simulink model "System_Design_Quadrocopter_Dynamics3"  (Simulink 7.4)
settings: Solver=ode45  StartTime=0.0  StopTime=inf  RelTol=1e-3
values from neighbouring files (symbols this model uses):
  K_ret = place(System.a, System.b, [-18 -10 -9 -5 -7])    [Test_Reglerauslegung.m]    (also in auslegung.m = place(System.a, System.b, [-2 -4 -3]))
  KV = KV'    [Reglerauslegung.m]    (also in Test_Reglerauslegung.m; auslegung.m)
  KvPhi = 0.5    [Test_Reglerauslegung.m]
  KvPsi = 0.08    [Test_Reglerauslegung.m]
  KvTheta = 0.4    [Test_Reglerauslegung.m]
undefined symbols (not defined in the file or in its folder): g, m, Ts
libraries: simulink x13, dspobslib x4, Control_lib x2, Copter_Library x1
(part 1 of 2)
settings Model: Creator=roczit00  LastModifiedBy=Mole
settings DebuggingCC: AlgebraicLoopMsg=none  SolverPrmCheckMsg=none  UnconnectedInputMsg=none  UnconnectedOutputMsg=none  UnconnectedLineMsg=none

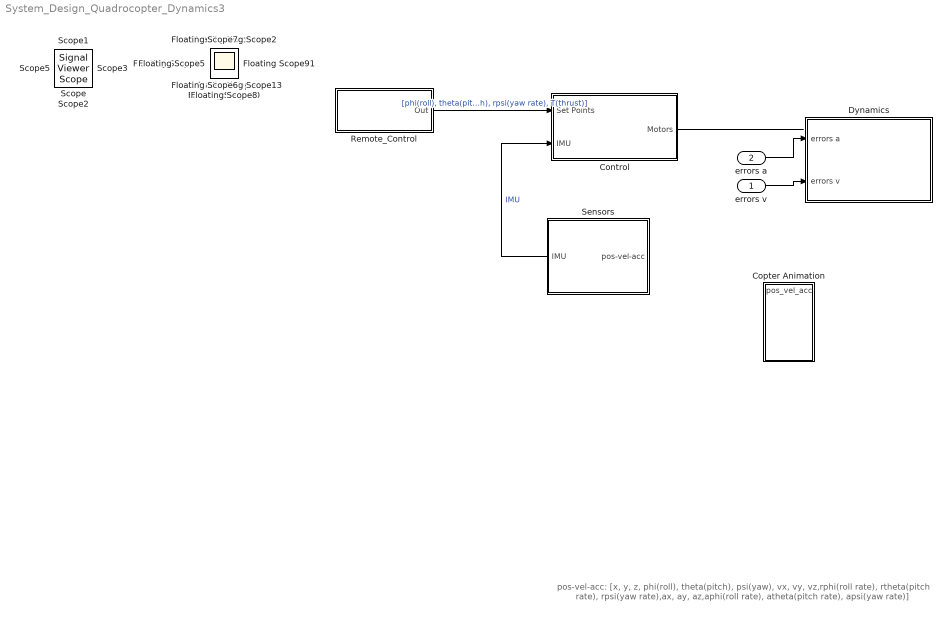
== system System_Design_Quadrocopter_Dynamics3 ==
  note: pos-vel-acc: [x, y, z, phi(roll), theta(pitch), psi(yaw), vx, vy, vz,rphi(roll rate), rtheta(pitch rate), rpsi(yaw rate),ax, ay, az,aphi(roll rate), atheta(pitch rate), apsi(yaw rate)]
  errors v : Inport
  errors a : Inport  Port=2
  Control : Subsystem
  Copter Animation : Subsystem  mask(Quadrocopter Animation){AXES=[-100 100 -100 100 0 100], T_INT=1/25, K_VAR=Feste Position, K_POS=[30 0 6], K_ANGLE=27, A_ON=on, u_phi=on, u_theta=on, u_psi=on, u_x=on, u_y=on, u_z=off}
      mask prompts: AXES "Achsen Grenzen [xmin xmax ymin ymax zmin zmax]"; T_INT "Zeitintervall zwischen Aktualisierungen [s]:"; K_VAR "Kamera Art:"; K_POS "Ort der Kamera [xc yc zc]:"; K_ANGLE "Öffnungswinkel der Kamera [Grad]:"; A_ON "Animation Einschalten:"; u_phi "Use Input phi:"; u_theta "Use Input theta:"; u_psi "Use Input psi:"; u_x "Use Input x:"; u_y "Use Input y:"; u_z "Use Input z:"
      mask help: Erstellt eine 3-D animierte Ansicht eines Quadrocopters.
      mask init:
      | Config.axes = AXES;
      | Config.update = T_INT;
      | Config.camera_view = K_VAR;
      | Config.camera_pos = K_POS;
      | Config.view = K_ANGLE;
      | Config.Animenable = A_ON;
      | Config.phi = u_phi;
      | Config.theta = u_theta;
      | Config.psi = u_psi;
      | Config.x = u_x;
      | Config.y = u_y;
      | Config.z = u_z;
      mask Help:
      | <p>Dieser Block erstellt ein 3 dimensionales Fenster eines Quadrocopters.
      | 
      | <p><H4>Block Eingänge</H4>
      | Der Eingangsvektor bestehend aus:
      | <ul>
      | <li>X-Koordinate - Ort bezogen auf die X-Achse
      | <li>Y-Koordinate - Ort bezogen auf die Y-Achse
      | <li>Z-Koordinate - Ort bezogen auf die Z-Achse
      | <li>Psi - Yaw Drehung um die Z-Achse
      | <li>Phi - Roll Drehen um die Achse in Flugrichtung
      | <li>theta - pitch Neigung in Flugrichtung nach oben bzw. unten
      | </ul></p>
      mask StyleString: edit,edit,popup(Feste Position|Frei bewegbar),edit,edit,checkbox,checkbox,checkbox,checkbox,checkbox,checkbox,checkbox
  Dynamics : Subsystem
  Remote_Control : Subsystem
  Sensors : Subsystem
  Floating Scope{,1..13} (14 alike) : Scope
      Floating Scope settings: Floating=on  YMin=-40  YMax=90
      Floating Scope1 settings: Floating=on
      Floating Scope10 settings: Floating=on  SaveName=ScopeData12
      Floating Scope11 settings: Floating=on  SaveName=ScopeData13
      Floating Scope12 settings: Floating=on  YMin=-2500  YMax=27500  SaveName=ScopeData14
      Floating Scope13 settings: Floating=on  YMin=0  YMax=0.3  SaveName=ScopeData15
      Floating Scope2 settings: Floating=on  YMin=-6000  YMax=2500  SaveName=ScopeData2
      Floating Scope3 settings: Floating=on  SaveName=ScopeData3
      Floating Scope4 settings: Floating=on  SaveName=ScopeData4
      Floating Scope5 settings: Floating=on  YMin=-0.7  YMax=0.8  SaveName=ScopeData5
      Floating Scope6 settings: Floating=on  YMin=-1  YMax=1  SaveName=ScopeData6
      Floating Scope7 settings: Floating=on  YMin=-15  YMax=10  SaveName=ScopeData7
      Floating Scope8 settings: Floating=on  YMax=45  SaveName=ScopeData10
      Floating Scope9 settings: Floating=on  YMin=-7  YMax=9  SaveName=ScopeData11
  Scope{,1..3,5} (5 alike) : SignalViewerScope  IOType=viewer  RefreshTime=0.035000
      Scope settings: YMin=-0.01  YMax=0.1
      Scope2 settings: SaveName=ScopeData2
      Scope3 settings: SaveName=ScopeData3
      Scope5 settings: YMin=0  YMax=275  SaveName=ScopeData4
  wires:
  ? -> Copter Animation/1(pos_vel_acc), Sensors/1(pos-vel-acc)  "pos-vel-acc"
  Sensors/1(IMU) -> Control/2(IMU)  "IMU"
  Remote_Control/1(Out) -> Control/1(Set Points)  "[phi(roll), theta(pitch), rpsi(yaw rate), T(thrust)]"
  errors v/1 -> Dynamics/2(errors v)
  Control/1(Motors) -> ?
  errors a/1 -> Dynamics/1(errors a)

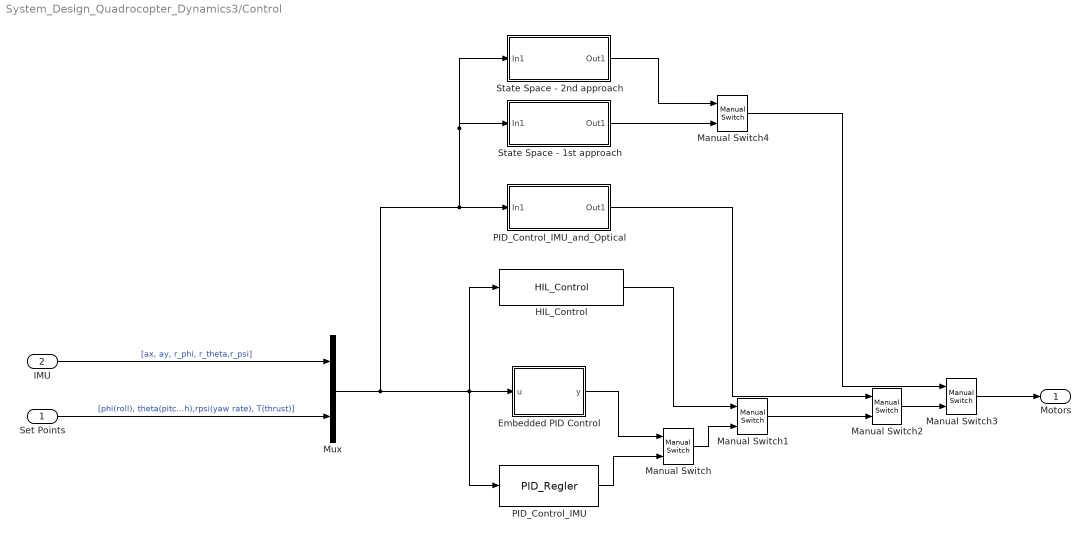
== system System_Design_Quadrocopter_Dynamics3/Control ==
  Set Points : Inport  PortDimensions=4  DataType=double  OutDataTypeStr=double
  IMU : Inport  Port=2
  Embedded PID Control : Stateflow chart  TreatAsAtomicUnit=on
  HIL_Control : Control_lib/HIL_Control  enabled=off
  Manual Switch{,2..4} (4 alike) : simulink/Signal Routing/Manual Switch  SystemSampleTime=-1  sw=1  action=0  varsize=off
  Manual Switch1 : simulink/Signal Routing/Manual Switch  SystemSampleTime=-1  sw=0  action=0  varsize=off
  Mux : Mux  Inputs=2
  PID_Control_IMU : Control_lib/PID_Regler  SystemSampleTime=-1
  PID_Control_IMU_and_Optical : Subsystem  AncestorBlock=Control_lib/PID_Regler
  State Space - 1st approach : Subsystem
  State Space - 2nd approach : Subsystem
  Motors : Outport  PortDimensions=4
  wires:
  IMU/1 -> Mux/1  "[ax, ay, r_phi, r_theta,r_psi]"
  Set Points/1 -> Mux/2  "[phi(roll), theta(pitch),rpsi(yaw rate), T(thrust)]"
  PID_Control_IMU/1 -> Manual Switch/2
  Mux/1 -> PID_Control_IMU/1, HIL_Control/1, Embedded PID Control/1(u), PID_Control_IMU_and_Optical/1(In1), State Space - 1st approach/1(In1), State Space - 2nd approach/1(In1)
  Manual Switch/1 -> Manual Switch1/2
  Manual Switch1/1 -> Manual Switch2/2
  Embedded PID Control/1(y) -> Manual Switch/1
  HIL_Control/1 -> Manual Switch1/1
  PID_Control_IMU_and_Optical/1(Out1) -> Manual Switch2/1
  Manual Switch2/1 -> Manual Switch3/2
  Manual Switch3/1 -> Motors/1
  Manual Switch4/1 -> Manual Switch3/1
  State Space - 1st approach/1(Out1) -> Manual Switch4/2
  State Space - 2nd approach/1(Out1) -> Manual Switch4/1

== system System_Design_Quadrocopter_Dynamics3/Copter Animation ==
  pos_vel_acc : Inport  PortDimensions=19
  S-Function : S-Function  FunctionName=Copter_Animation  Parameters=Config  EnableBusSupport=off
  Selector2 : Selector  InputPortWidth=19  IndexOptions=Index vector (dialog)  Indices=[1 2 3 4 5 6]  OutputSizes=1
  wires:
  pos_vel_acc/1 -> Selector2/1
  Selector2/1 -> S-Function/1

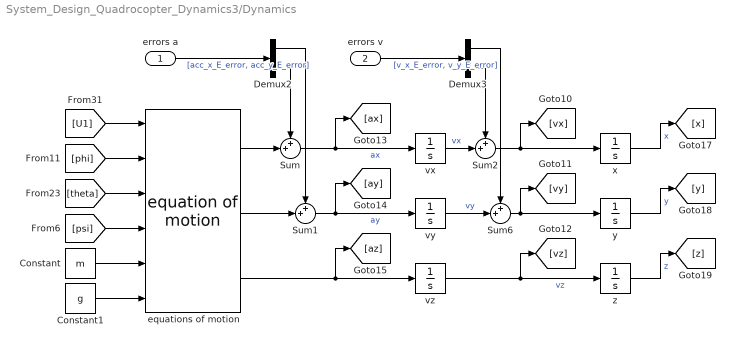
== system System_Design_Quadrocopter_Dynamics3/Dynamics ==
  errors a : Inport
  errors v : Inport  Port=2
  Constant : Constant  Value=m
  Constant1 : Constant  Value=g
  Demux2 : Demux  Outputs=2
  Demux3 : Demux  Outputs=2
  Sum{,1..2,6} (4 alike) : Sum  Inputs=++|
  equations of motion : Copter_Library/equation of motion  SystemSampleTime=-1
  vx : Integrator
  vy : Integrator
  vz : Integrator
  x : Integrator
  y : Integrator
  z : Integrator
  wires:
  errors a/1 -> Demux2/1  "[acc_x_E_error, acc_y_E_error]"
  vz/1 -> [vz], z/1  "vz"
  Demux2/2 -> Sum/1
  Demux2/1 -> Sum1/1
  equations of motion/3 -> [az], vz/1
  equations of motion/2 -> Sum1/2
  equations of motion/1 -> Sum/2
  [phi] -> equations of motion/2
  [theta] -> equations of motion/3
  [psi] -> equations of motion/4
  Constant/1 -> equations of motion/5
  Constant1/1 -> equations of motion/6
  errors v/1 -> Demux3/1  "[v_x_E_error, v_y_E_error]"
  Demux3/2 -> Sum2/1
  Demux3/1 -> Sum6/1
  vx/1 -> Sum2/2  "vx"
  Sum2/1 -> [vx], x/1
  vy/1 -> Sum6/2  "vy"
  Sum6/1 -> y/1, [vy]
  z/1 -> [z]  "z"
  y/1 -> [y]  "y"
  x/1 -> [x]  "x"
  Sum1/1 -> vy/1, [ay]  "ay"
  Sum/1 -> vx/1, [ax]  "ax"
  [U1] -> equations of motion/1

== system System_Design_Quadrocopter_Dynamics3/Remote_Control ==
  3D-Mouse : simulink/Signal Routing/Manual Switch  SystemSampleTime=-1  sw=0  action=0  varsize=off
  Allow 3D Mouse : dspobslib/DSP Constant  SystemSampleTime=-1  Value=1  SampleMode=Discrete  discreteOutput=Sample-based  continuousOutput=Sample-based  sampTime=inf  framePeriod=2  dataType=boolean  isSigned=on  wordLen=16  udDataType=sfix(16)  fracBitsMode=Best precision  numFracBits=15  InterpretAs1D=-inf  Ts=-inf  FramebasedOutput=-inf
  Disable 3D Mouse : dspobslib/DSP Constant  SystemSampleTime=-1  Value=0  SampleMode=Discrete  discreteOutput=Sample-based  continuousOutput=Sample-based  sampTime=inf  framePeriod=2  dataType=boolean  isSigned=on  wordLen=16  udDataType=sfix(16)  fracBitsMode=Best precision  numFracBits=15  InterpretAs1D=-inf  Ts=-inf  FramebasedOutput=-inf
  Manual Switch2 : simulink/Signal Routing/Manual Switch  SystemSampleTime=-1  sw=1  action=0  varsize=off
  Remote_Control_3d_mouse : Subsystem  AncestorBlock=Remote_Control_Library/Remote_Control_3d_mouse
  Remote_Control_Pitch_stimuli1 : Subsystem  AncestorBlock=Remote_Control_Library/Remote_Control_Pitch_stimuli
  Out : Outport
  wires:
  Remote_Control_Pitch_stimuli1/1(Out) -> Manual Switch2/1
  Manual Switch2/1 -> Out/1
  Allow 3D Mouse/1 -> 3D-Mouse/1
  Disable 3D Mouse/1 -> 3D-Mouse/2
  3D-Mouse/1 -> Remote_Control_3d_mouse/Enable
  Remote_Control_3d_mouse/1(Out1) -> Manual Switch2/2

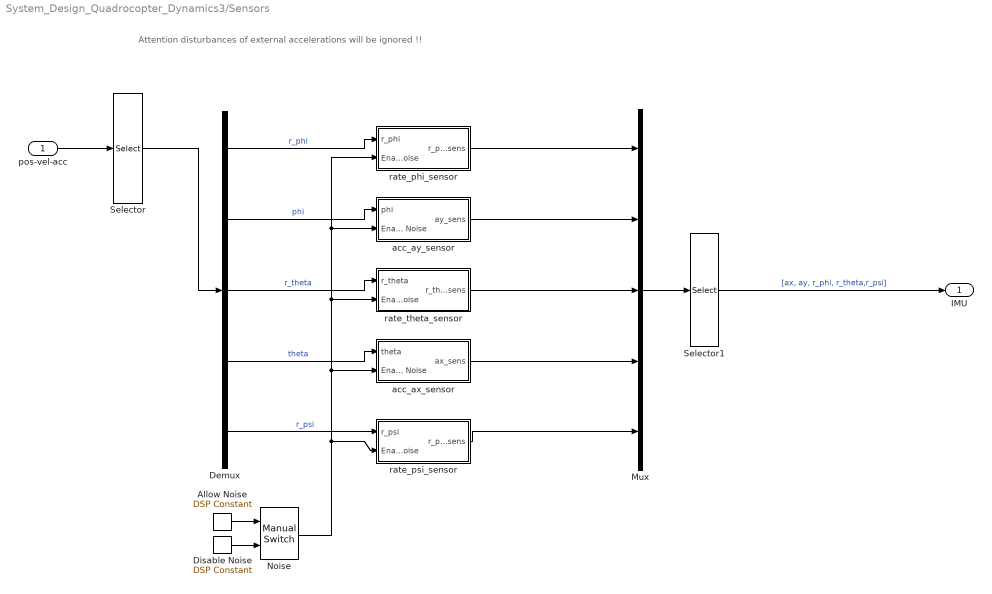
== system System_Design_Quadrocopter_Dynamics3/Sensors ==
  note: Attention disturbances of external accelerations will be ignored !!
  pos-vel-acc : Inport  PortDimensions=19
  Allow Noise : dspobslib/DSP Constant  SystemSampleTime=-1  Value=1  SampleMode=Discrete  discreteOutput=Sample-based  continuousOutput=Sample-based  sampTime=inf  framePeriod=2  dataType=boolean  isSigned=on  wordLen=16  udDataType=sfix(16)  fracBitsMode=Best precision  numFracBits=15  InterpretAs1D=-inf  Ts=-inf  FramebasedOutput=-inf
  Demux : Demux  Outputs=5
  Disable Noise : dspobslib/DSP Constant  SystemSampleTime=-1  Value=0  SampleMode=Discrete  discreteOutput=Sample-based  continuousOutput=Sample-based  sampTime=inf  framePeriod=2  dataType=boolean  isSigned=on  wordLen=16  udDataType=sfix(16)  fracBitsMode=Best precision  numFracBits=15  InterpretAs1D=-inf  Ts=-inf  FramebasedOutput=-inf
  Mux : Mux  Inputs=5
  Noise : simulink/Signal Routing/Manual Switch  SystemSampleTime=-1  sw=1  action=0  varsize=off
  Selector : Selector  InputPortWidth=19  IndexOptions=Index vector (dialog)  Indices=[10 4 11 5 12]  OutputSizes=1
  Selector1 : Selector  InputPortWidth=5  IndexOptions=Index vector (dialog)  Indices=[4 2 1 3 5]  OutputSizes=1
  acc_ax_sensor : Subsystem
  acc_ay_sensor : Subsystem
  rate_phi_sensor : Subsystem
  rate_psi_sensor : Subsystem
  rate_theta_sensor : Subsystem
  IMU : Outport
  wires:
  pos-vel-acc/1 -> Selector/1
  Selector/1 -> Demux/1
  rate_phi_sensor/1(r_phi_sens) -> Mux/1
  acc_ay_sensor/1(ay_sens) -> Mux/2
  rate_theta_sensor/1(r_theta_sens) -> Mux/3
  acc_ax_sensor/1(ax_sens) -> Mux/4
  rate_psi_sensor/1(r_psi_sens) -> Mux/5
  Demux/1 -> rate_phi_sensor/1(r_phi)  "r_phi"
  Demux/2 -> acc_ay_sensor/1(phi)  "phi"
  Demux/3 -> rate_theta_sensor/1(r_theta)  "r_theta"
  Demux/4 -> acc_ax_sensor/1(theta)  "theta"
  Demux/5 -> rate_psi_sensor/1(r_psi)  "r_psi"
  Mux/1 -> Selector1/1
  Selector1/1 -> IMU/1  "[ax, ay, r_phi, r_theta,r_psi]"
  Allow Noise/1 -> Noise/1
  Disable Noise/1 -> Noise/2
  Noise/1 -> rate_psi_sensor/2(Enable Noise), acc_ax_sensor/2(Enable Noise), rate_theta_sensor/2(Enable Noise), acc_ay_sensor/2(Enable Noise), rate_phi_sensor/2(Enable Noise)

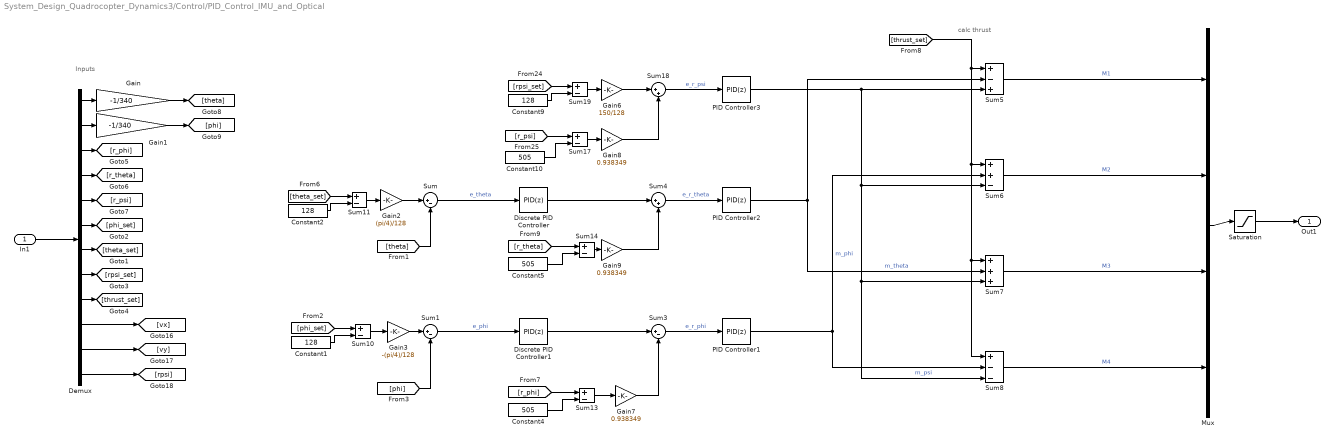
== system System_Design_Quadrocopter_Dynamics3/Control/PID_Control_IMU_and_Optical ==
  note: calc thrust
  note: Inputs
  In1 : Inport  OutDataType=fixdt(1, 16)  OutScaling=2^0
  Constant1 : Constant  Value=128  OutDataType=fixdt(1, 16)  OutScaling=2^0
  Constant10 : Constant  Value=505  OutDataType=fixdt(1, 16)  OutScaling=2^0
  Constant2 : Constant  Value=128  OutDataType=fixdt(1, 16)  OutScaling=2^0
  Constant4 : Constant  Value=505  OutDataType=fixdt(1, 16)  OutScaling=2^0
  Constant5 : Constant  Value=505  OutDataType=fixdt(1, 16)  OutScaling=2^0
  Constant9 : Constant  Value=128  OutDataType=fixdt(1, 16)  OutScaling=2^0
  Demux : Demux  Outputs=12
  Discrete PID Controller : simulink/Continuous/PID Controller  DialogController=pidpack.PIDConfig.pidDDGCreate  DialogControllerArgs=DataTag0  SystemSampleTime=-1  Controller=PID  TimeDomain=Discrete-time  SampleTime=Ts  IntegratorMethod=Forward Euler  FilterMethod=Forward Euler  Form=Ideal  P=150  I=0.5  D=0  N=0  InitialConditionSource=internal  InitialConditionForIntegrator=0  InitialConditionForFilter=0  ExternalReset=none  ZeroCross=off  LimitOutput=off  UpperSaturationLimit=inf  LowerSaturationLimit=-inf  LinearizeAsGain=off  AntiWindupMode=none  Kb=1  TrackingMode=off  Kt=1  PParamMin=[]  PParamMax=[]  IParamMin=[]  IParamMax=[]  DParamMin=[]  DParamMax=[]  NParamMin=[]  NParamMax=[]  KbParamMin=[]  KbParamMax=[]  KtParamMin=[]  KtParamMax=[]  POutMin=[]  POutMax=[]  IOutMin=[]  IOutMax=[]  DOutMin=[]  DOutMax=[]  NOutMin=[]  NOutMax=[]  KbOutMin=[]  KbOutMax=[]  KtOutMin=[]  KtOutMax=[]  IntegratorOutMin=[]  IntegratorOutMax=[]  FilterOutMin=[]  FilterOutMax=[]  SumOutMin=[]  SumOutMax=[]  SumI1OutMin=[]  SumI1OutMax=[]  SumI2OutMin=[]  SumI2OutMax=[]  SumI3OutMin=[]  SumI3OutMax=[]  SumDOutMin=[]  SumDOutMax=[]  SaturationOutMin=[]  SaturationOutMax=[]  IntegratorContinuousStateAttributes=''  IntegratorStateMustResolveToSignalObject=off  IntegratorRTWStateStorageClass=Auto  FilterContinuousStateAttributes=''  FilterStateMustResolveToSignalObject=off  FilterRTWStateStorageClass=Auto
  Discrete PID Controller1 : simulink/Continuous/PID Controller  DialogController=pidpack.PIDConfig.pidDDGCreate  DialogControllerArgs=DataTag1  SystemSampleTime=-1  Controller=PID  TimeDomain=Discrete-time  SampleTime=Ts  IntegratorMethod=Forward Euler  FilterMethod=Forward Euler  Form=Ideal  P=150  I=0.5  D=0  N=0  InitialConditionSource=internal  InitialConditionForIntegrator=0  InitialConditionForFilter=0  ExternalReset=none  ZeroCross=off  LimitOutput=off  UpperSaturationLimit=inf  LowerSaturationLimit=-inf  LinearizeAsGain=off  AntiWindupMode=none  Kb=1  TrackingMode=off  Kt=1  PParamMin=[]  PParamMax=[]  IParamMin=[]  IParamMax=[]  DParamMin=[]  DParamMax=[]  NParamMin=[]  NParamMax=[]  KbParamMin=[]  KbParamMax=[]  KtParamMin=[]  KtParamMax=[]  POutMin=[]  POutMax=[]  IOutMin=[]  IOutMax=[]  DOutMin=[]  DOutMax=[]  NOutMin=[]  NOutMax=[]  KbOutMin=[]  KbOutMax=[]  KtOutMin=[]  KtOutMax=[]  IntegratorOutMin=[]  IntegratorOutMax=[]  FilterOutMin=[]  FilterOutMax=[]  SumOutMin=[]  SumOutMax=[]  SumI1OutMin=[]  SumI1OutMax=[]  SumI2OutMin=[]  SumI2OutMax=[]  SumI3OutMin=[]  SumI3OutMax=[]  SumDOutMin=[]  SumDOutMax=[]  SaturationOutMin=[]  SaturationOutMax=[]  IntegratorContinuousStateAttributes=''  IntegratorStateMustResolveToSignalObject=off  IntegratorRTWStateStorageClass=Auto  FilterContinuousStateAttributes=''  FilterStateMustResolveToSignalObject=off  FilterRTWStateStorageClass=Auto
  Gain : Gain  Gain=-1/340  ParameterDataType=fixdt(1, 16)  ParameterScaling=2^0  OutDataType=fixdt(1, 16)  OutScaling=2^0
  Gain1 : Gain  Gain=-1/340  ParameterDataType=fixdt(1, 16)  ParameterScaling=2^0  OutDataType=fixdt(1, 16)  OutScaling=2^0
  Gain2 : Gain  Gain=(pi/4)/128  ParameterDataType=fixdt(1, 16)  ParameterScaling=2^0  OutDataType=fixdt(1, 16)  OutScaling=2^0
  Gain3 : Gain  Gain=-(pi/4)/128  ParameterDataType=fixdt(1, 16)  ParameterScaling=2^0  OutDataType=fixdt(1, 16)  OutScaling=2^0
  Gain6 : Gain  Gain=150/128  ParameterDataType=fixdt(1, 16)  ParameterScaling=2^0  OutDataType=fixdt(1, 16)  OutScaling=2^0
  Gain7 : Gain  Gain=0.938349  ParameterDataType=fixdt(1, 16)  ParameterScaling=2^0  OutDataType=fixdt(1, 16)  OutScaling=2^0
  Gain8 : Gain  Gain=0.938349  ParameterDataType=fixdt(1, 16)  ParameterScaling=2^0  OutDataType=fixdt(1, 16)  OutScaling=2^0
  Gain9 : Gain  Gain=0.938349  ParameterDataType=fixdt(1, 16)  ParameterScaling=2^0  OutDataType=fixdt(1, 16)  OutScaling=2^0
  Mux : Mux
  PID Controller1 : simulink/Continuous/PID Controller  DialogController=pidpack.PIDConfig.pidDDGCreate  DialogControllerArgs=DataTag2  SystemSampleTime=-1  Controller=PID  TimeDomain=Discrete-time  SampleTime=Ts  IntegratorMethod=Forward Euler  FilterMethod=Forward Euler  Form=Ideal  P=60  I=0.5  D=0  N=0  InitialConditionSource=internal  InitialConditionForIntegrator=0  InitialConditionForFilter=0  ExternalReset=none  ZeroCross=off  LimitOutput=off  UpperSaturationLimit=inf  LowerSaturationLimit=-inf  LinearizeAsGain=off  AntiWindupMode=none  Kb=1  TrackingMode=off  Kt=1  PParamMin=[]  PParamMax=[]  IParamMin=[]  IParamMax=[]  DParamMin=[]  DParamMax=[]  NParamMin=[]  NParamMax=[]  KbParamMin=[]  KbParamMax=[]  KtParamMin=[]  KtParamMax=[]  POutMin=[]  POutMax=[]  IOutMin=[]  IOutMax=[]  DOutMin=[]  DOutMax=[]  NOutMin=[]  NOutMax=[]  KbOutMin=[]  KbOutMax=[]  KtOutMin=[]  KtOutMax=[]  IntegratorOutMin=[]  IntegratorOutMax=[]  FilterOutMin=[]  FilterOutMax=[]  SumOutMin=[]  SumOutMax=[]  SumI1OutMin=[]  SumI1OutMax=[]  SumI2OutMin=[]  SumI2OutMax=[]  SumI3OutMin=[]  SumI3OutMax=[]  SumDOutMin=[]  SumDOutMax=[]  SaturationOutMin=[]  SaturationOutMax=[]  IntegratorContinuousStateAttributes=''  IntegratorStateMustResolveToSignalObject=off  IntegratorRTWStateStorageClass=Auto  FilterContinuousStateAttributes=''  FilterStateMustResolveToSignalObject=off  FilterRTWStateStorageClass=Auto
  PID Controller2 : simulink/Continuous/PID Controller  DialogController=pidpack.PIDConfig.pidDDGCreate  DialogControllerArgs=DataTag3  SystemSampleTime=-1  Controller=PID  TimeDomain=Discrete-time  SampleTime=Ts  IntegratorMethod=Forward Euler  FilterMethod=Forward Euler  Form=Ideal  P=60  I=0.5  D=0  N=0  InitialConditionSource=internal  InitialConditionForIntegrator=0  InitialConditionForFilter=0  ExternalReset=none  ZeroCross=off  LimitOutput=off  UpperSaturationLimit=inf  LowerSaturationLimit=-inf  LinearizeAsGain=off  AntiWindupMode=none  Kb=1  TrackingMode=off  Kt=1  PParamMin=[]  PParamMax=[]  IParamMin=[]  IParamMax=[]  DParamMin=[]  DParamMax=[]  NParamMin=[]  NParamMax=[]  KbParamMin=[]  KbParamMax=[]  KtParamMin=[]  KtParamMax=[]  POutMin=[]  POutMax=[]  IOutMin=[]  IOutMax=[]  DOutMin=[]  DOutMax=[]  NOutMin=[]  NOutMax=[]  KbOutMin=[]  KbOutMax=[]  KtOutMin=[]  KtOutMax=[]  IntegratorOutMin=[]  IntegratorOutMax=[]  FilterOutMin=[]  FilterOutMax=[]  SumOutMin=[]  SumOutMax=[]  SumI1OutMin=[]  SumI1OutMax=[]  SumI2OutMin=[]  SumI2OutMax=[]  SumI3OutMin=[]  SumI3OutMax=[]  SumDOutMin=[]  SumDOutMax=[]  SaturationOutMin=[]  SaturationOutMax=[]  IntegratorContinuousStateAttributes=''  IntegratorStateMustResolveToSignalObject=off  IntegratorRTWStateStorageClass=Auto  FilterContinuousStateAttributes=''  FilterStateMustResolveToSignalObject=off  FilterRTWStateStorageClass=Auto
  PID Controller3 : simulink/Continuous/PID Controller  DialogController=pidpack.PIDConfig.pidDDGCreate  DialogControllerArgs=DataTag4  SystemSampleTime=-1  Controller=PID  TimeDomain=Discrete-time  SampleTime=Ts  IntegratorMethod=Forward Euler  FilterMethod=Forward Euler  Form=Ideal  P=60  I=0.5  D=0  N=0  InitialConditionSource=internal  InitialConditionForIntegrator=0  InitialConditionForFilter=0  ExternalReset=none  ZeroCross=off  LimitOutput=off  UpperSaturationLimit=inf  LowerSaturationLimit=-inf  LinearizeAsGain=off  AntiWindupMode=none  Kb=1  TrackingMode=off  Kt=1  PParamMin=[]  PParamMax=[]  IParamMin=[]  IParamMax=[]  DParamMin=[]  DParamMax=[]  NParamMin=[]  NParamMax=[]  KbParamMin=[]  KbParamMax=[]  KtParamMin=[]  KtParamMax=[]  POutMin=[]  POutMax=[]  IOutMin=[]  IOutMax=[]  DOutMin=[]  DOutMax=[]  NOutMin=[]  NOutMax=[]  KbOutMin=[]  KbOutMax=[]  KtOutMin=[]  KtOutMax=[]  IntegratorOutMin=[]  IntegratorOutMax=[]  FilterOutMin=[]  FilterOutMax=[]  SumOutMin=[]  SumOutMax=[]  SumI1OutMin=[]  SumI1OutMax=[]  SumI2OutMin=[]  SumI2OutMax=[]  SumI3OutMin=[]  SumI3OutMax=[]  SumDOutMin=[]  SumDOutMax=[]  SaturationOutMin=[]  SaturationOutMax=[]  IntegratorContinuousStateAttributes=''  IntegratorStateMustResolveToSignalObject=off  IntegratorRTWStateStorageClass=Auto  FilterContinuousStateAttributes=''  FilterStateMustResolveToSignalObject=off  FilterRTWStateStorageClass=Auto
  Saturation : Saturate  UpperLimit=255  LowerLimit=0  OutDataType=fixdt(1, 16)  OutScaling=2^0
  Sum : Sum  Inputs=|+-  OutDataType=fixdt(1, 16)  OutScaling=2^0
  Sum1 : Sum  Inputs=|+-  OutDataType=fixdt(1, 16)  OutScaling=2^0
  Sum{10..11,13..14,17,19} (6 alike) : Sum  Inputs=+-  OutDataType=fixdt(1, 16)  OutScaling=2^0
  Sum18 : Sum  Inputs=|++  OutDataType=fixdt(1, 16)  OutScaling=2^0
  Sum3 : Sum  Inputs=|+-  OutDataType=fixdt(1, 16)  OutScaling=2^0
  Sum4 : Sum  Inputs=|++  OutDataType=fixdt(1, 16)  OutScaling=2^0
  Sum5 : Sum  Inputs=+-+  OutDataType=fixdt(1, 16)  OutScaling=2^0
  Sum6 : Sum  Inputs=++-  OutDataType=fixdt(1, 16)  OutScaling=2^0
  Sum7 : Sum  Inputs=+++  OutDataType=fixdt(1, 16)  OutScaling=2^0
  Sum8 : Sum  Inputs=+--  OutDataType=fixdt(1, 16)  OutScaling=2^0
  Out1 : Outport  OutDataType=fixdt(1, 16)  OutScaling=2^0
  wires:
  Sum14/1 -> Gain9/1
  Gain9/1 -> Sum4/2
  Sum13/1 -> Gain7/1
  Gain3/1 -> Sum1/1
  Gain2/1 -> Sum/1
  Sum11/1 -> Gain2/1
  Sum10/1 -> Gain3/1
  [r_theta] -> Sum14/1
  Constant5/1 -> Sum14/2
  [r_phi] -> Sum13/1
  Constant4/1 -> Sum13/2
  Constant2/1 -> Sum11/2
  [theta_set] -> Sum11/1
  Constant1/1 -> Sum10/2
  [phi_set] -> Sum10/1
  Saturation/1 -> Out1/1
  Mux/1 -> Saturation/1
  [thrust_set] -> Sum8/1, Sum7/1, Sum6/1, Sum5/1
  PID Controller1/1 -> Sum6/2, Sum8/2  "m_phi"
  Sum6/1 -> Mux/2  "M2"
  Sum7/1 -> Mux/3  "M3"
  Sum8/1 -> Mux/4  "M4"
  Sum5/1 -> Mux/1  "M1"
  Sum4/1 -> PID Controller2/1  "e_r_theta"
  Sum3/1 -> PID Controller1/1  "e_r_phi"
  Sum1/1 -> Discrete PID Controller1/1  "e_phi"
  [phi] -> Sum1/2
  Sum/1 -> Discrete PID Controller/1  "e_theta"
  [theta] -> Sum/2
  Gain1/1 -> [phi]
  Gain/1 -> [theta]
  Demux/9 -> [thrust_set]
  Demux/8 -> [rpsi_set]
  Demux/7 -> [theta_set]
  Demux/6 -> [phi_set]
  Demux/5 -> [r_psi]
  Demux/4 -> [r_theta]
  Demux/3 -> [r_phi]
  Demux/1 -> Gain/1
  Demux/2 -> Gain1/1
  In1/1 -> Demux/1
  Demux/10 -> [vx]
  Demux/11 -> [vy]
  Demux/12 -> [rpsi]
  Gain8/1 -> Sum18/2
  Sum17/1 -> Gain8/1
  Gain6/1 -> Sum18/1
  Sum19/1 -> Gain6/1
  Constant10/1 -> Sum17/2
  [r_psi] -> Sum17/1
  Constant9/1 -> Sum19/2
  [rpsi_set] -> Sum19/1
  Sum18/1 -> PID Controller3/1  "e_r_psi"
  Discrete PID Controller1/1 -> Sum3/1
  Discrete PID Controller/1 -> Sum4/1
  Gain7/1 -> Sum3/2
  PID Controller3/1 -> Sum5/3, Sum6/3, Sum7/3, Sum8/3  "m_psi"
  PID Controller2/1 -> Sum7/2, Sum5/2  "m_theta"

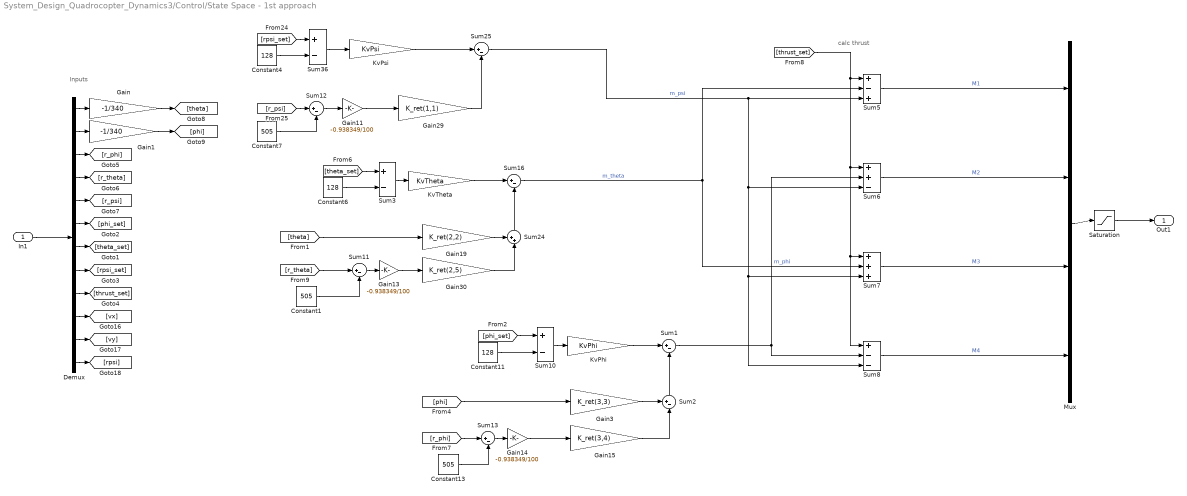
== system System_Design_Quadrocopter_Dynamics3/Control/State Space - 1st approach ==
  note: calc thrust
  note: Inputs
  In1 : Inport  OutDataType=fixdt(1, 16)  OutScaling=2^0
  Constant1 : Constant  Value=505  OutDataType=fixdt(1, 16)  OutScaling=2^0
  Constant11 : Constant  Value=128  OutDataType=fixdt(1, 16)  OutScaling=2^0
  Constant13 : Constant  Value=505  OutDataType=fixdt(1, 16)  OutScaling=2^0
  Constant4 : Constant  Value=128  OutDataType=fixdt(1, 16)  OutScaling=2^0
  Constant6 : Constant  Value=128  OutDataType=fixdt(1, 16)  OutScaling=2^0
  Constant7 : Constant  Value=505  OutDataType=fixdt(1, 16)  OutScaling=2^0
  Demux : Demux  Outputs=12
  Gain : Gain  Gain=-1/340  ParameterDataType=fixdt(1, 16)  ParameterScaling=2^0  OutDataType=fixdt(1, 16)  OutScaling=2^0
  Gain1 : Gain  Gain=-1/340  ParameterDataType=fixdt(1, 16)  ParameterScaling=2^0  OutDataType=fixdt(1, 16)  OutScaling=2^0
  Gain11 : Gain  Gain=-0.938349/100  ParameterDataType=fixdt(1, 16)  ParameterScaling=2^0  OutDataType=fixdt(1, 16)  OutScaling=2^0
  Gain13 : Gain  Gain=-0.938349/100  ParameterDataType=fixdt(1, 16)  ParameterScaling=2^0  OutDataType=fixdt(1, 16)  OutScaling=2^0
  Gain14 : Gain  Gain=-0.938349/100  ParameterDataType=fixdt(1, 16)  ParameterScaling=2^0  OutDataType=fixdt(1, 16)  OutScaling=2^0
  Gain15 : Gain  Gain=K_ret(3,4)  ParameterDataType=fixdt(1, 16)  ParameterScaling=2^0  OutDataType=fixdt(1, 16)  OutScaling=2^0
  Gain19 : Gain  Gain=K_ret(2,2)  ParameterDataType=fixdt(1, 16)  ParameterScaling=2^0  OutDataType=fixdt(1, 16)  OutScaling=2^0
  Gain29 : Gain  Gain=K_ret(1,1)  ParameterDataType=fixdt(1, 16)  ParameterScaling=2^0  OutDataType=fixdt(1, 16)  OutScaling=2^0
  Gain3 : Gain  Gain=K_ret(3,3)  ParameterDataType=fixdt(1, 16)  ParameterScaling=2^0  OutDataType=fixdt(1, 16)  OutScaling=2^0
  Gain30 : Gain  Gain=K_ret(2,5)  ParameterDataType=fixdt(1, 16)  ParameterScaling=2^0  OutDataType=fixdt(1, 16)  OutScaling=2^0
  KvPhi : Gain  Gain=KvPhi  ParameterDataType=fixdt(1, 16)  ParameterScaling=2^0  OutDataType=fixdt(1, 16)  OutScaling=2^0
  KvPsi : Gain  Gain=KvPsi  ParameterDataType=fixdt(1, 16)  ParameterScaling=2^0  OutDataType=fixdt(1, 16)  OutScaling=2^0
  KvTheta : Gain  Gain=KvTheta  ParameterDataType=fixdt(1, 16)  ParameterScaling=2^0  OutDataType=fixdt(1, 16)  OutScaling=2^0
  Mux : Mux
  Saturation : Saturate  UpperLimit=255  LowerLimit=0  OutDataType=fixdt(1, 16)  OutScaling=2^0
  Sum{1,11..13,16,25} (6 alike) : Sum  Inputs=|+-  OutDataType=fixdt(1, 16)  OutScaling=2^0
  Sum10 : Sum  Inputs=+-  OutDataType=fixdt(1, 16)  OutScaling=2^0
  Sum2 : Sum  Inputs=+-|  OutDataType=fixdt(1, 16)  OutScaling=2^0
  Sum24 : Sum  Inputs=++|  OutDataType=fixdt(1, 16)  OutScaling=2^0
  Sum3 : Sum  Inputs=+-  OutDataType=fixdt(1, 16)  OutScaling=2^0
  Sum36 : Sum  Inputs=+-  OutDataType=fixdt(1, 16)  OutScaling=2^0
  Sum5 : Sum  Inputs=+-+  OutDataType=fixdt(1, 16)  OutScaling=2^0
  Sum6 : Sum  Inputs=++-  OutDataType=fixdt(1, 16)  OutScaling=2^0
  Sum7 : Sum  Inputs=+++  OutDataType=fixdt(1, 16)  OutScaling=2^0
  Sum8 : Sum  Inputs=+--  OutDataType=fixdt(1, 16)  OutScaling=2^0
  Out1 : Outport  OutDataType=fixdt(1, 16)  OutScaling=2^0
  wires:
  Saturation/1 -> Out1/1
  Mux/1 -> Saturation/1
  [thrust_set] -> Sum8/1, Sum7/1, Sum6/1, Sum5/1
  Sum1/1 -> Sum6/2, Sum8/2  "m_phi"
  Sum6/1 -> Mux/2  "M2"
  Sum7/1 -> Mux/3  "M3"
  Sum8/1 -> Mux/4  "M4"
  Sum5/1 -> Mux/1  "M1"
  Gain1/1 -> [phi]
  Gain/1 -> [theta]
  Demux/9 -> [thrust_set]
  Demux/8 -> [rpsi_set]
  Demux/7 -> [theta_set]
  Demux/6 -> [phi_set]
  Demux/5 -> [r_psi]
  Demux/4 -> [r_theta]
  Demux/3 -> [r_phi]
  Demux/1 -> Gain/1
  Demux/2 -> Gain1/1
  In1/1 -> Demux/1
  Demux/10 -> [vx]
  Demux/11 -> [vy]
  Demux/12 -> [rpsi]
  Sum25/1 -> Sum5/3, Sum6/3, Sum7/3, Sum8/3  "m_psi"
  Sum16/1 -> Sum7/2, Sum5/2  "m_theta"
  Sum2/1 -> Sum1/2
  [r_phi] -> Sum13/1
  Sum10/1 -> KvPhi/1
  Gain3/1 -> Sum2/1
  [phi] -> Gain3/1
  Sum13/1 -> Gain14/1
  Constant13/1 -> Sum13/2
  Gain14/1 -> Gain15/1
  Gain15/1 -> Sum2/2
  KvPhi/1 -> Sum1/1
  Constant11/1 -> Sum10/2
  [phi_set] -> Sum10/1
  KvTheta/1 -> Sum16/1
  Sum24/1 -> Sum16/2
  Sum3/1 -> KvTheta/1
  Gain30/1 -> Sum24/2
  Gain19/1 -> Sum24/1
  [theta] -> Gain19/1
  Gain13/1 -> Gain30/1
  Sum11/1 -> Gain13/1
  Constant1/1 -> Sum11/2
  [r_theta] -> Sum11/1
  [theta_set] -> Sum3/1
  Constant6/1 -> Sum3/2
  KvPsi/1 -> Sum25/1
  Gain29/1 -> Sum25/2
  Sum36/1 -> KvPsi/1
  Gain11/1 -> Gain29/1
  Sum12/1 -> Gain11/1
  [r_psi] -> Sum12/1
  Constant4/1 -> Sum36/2
  [rpsi_set] -> Sum36/1
  Constant7/1 -> Sum12/2

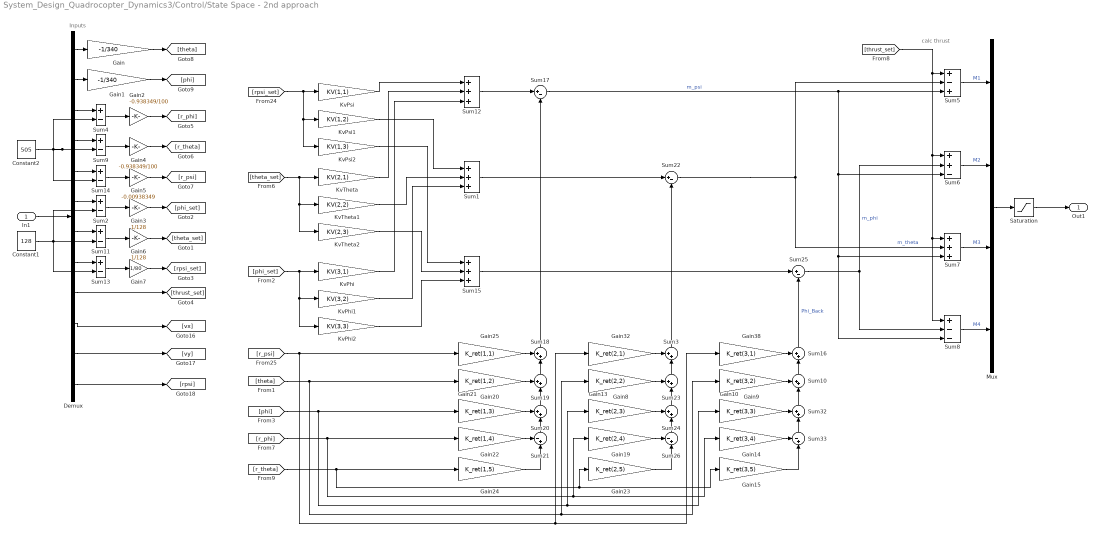
== system System_Design_Quadrocopter_Dynamics3/Control/State Space - 2nd approach ==
  note: calc thrust
  note: Inputs
  In1 : Inport  OutDataType=fixdt(1, 16)  OutScaling=2^0
  Constant1 : Constant  Value=128  OutDataType=fixdt(1, 16)  OutScaling=2^0
  Constant2 : Constant  Value=505  OutDataType=fixdt(1, 16)  OutScaling=2^0
  Demux : Demux  Outputs=12
  Gain : Gain  Gain=-1/340  ParameterDataType=fixdt(1, 16)  ParameterScaling=2^0  OutDataType=fixdt(1, 16)  OutScaling=2^0
  Gain1 : Gain  Gain=-1/340  ParameterDataType=fixdt(1, 16)  ParameterScaling=2^0  OutDataType=fixdt(1, 16)  OutScaling=2^0
  Gain10 : Gain  Gain=K_ret(3,3)  ParameterDataType=fixdt(1, 16)  ParameterScaling=2^0  OutDataType=fixdt(1, 16)  OutScaling=2^0
  Gain13 : Gain  Gain=K_ret(2,3)  ParameterDataType=fixdt(1, 16)  ParameterScaling=2^0  OutDataType=fixdt(1, 16)  OutScaling=2^0
  Gain14 : Gain  Gain=K_ret(3,4)  ParameterDataType=fixdt(1, 16)  ParameterScaling=2^0  OutDataType=fixdt(1, 16)  OutScaling=2^0
  Gain15 : Gain  Gain=K_ret(3,5)  ParameterDataType=fixdt(1, 16)  ParameterScaling=2^0  OutDataType=fixdt(1, 16)  OutScaling=2^0
  Gain19 : Gain  Gain=K_ret(2,4)  ParameterDataType=fixdt(1, 16)  ParameterScaling=2^0  OutDataType=fixdt(1, 16)  OutScaling=2^0
  Gain2 : Gain  Gain=-0.938349/100  ParameterDataType=fixdt(1, 16)  ParameterScaling=2^0  OutDataType=fixdt(1, 16)  OutScaling=2^0
  Gain20 : Gain  Gain=K_ret(1,2)  ParameterDataType=fixdt(1, 16)  ParameterScaling=2^0  OutDataType=fixdt(1, 16)  OutScaling=2^0
  Gain21 : Gain  Gain=K_ret(1,3)  ParameterDataType=fixdt(1, 16)  ParameterScaling=2^0  OutDataType=fixdt(1, 16)  OutScaling=2^0
  Gain22 : Gain  Gain=K_ret(1,4)  ParameterDataType=fixdt(1, 16)  ParameterScaling=2^0  OutDataType=fixdt(1, 16)  OutScaling=2^0
  Gain23 : Gain  Gain=K_ret(2,5)  ParameterDataType=fixdt(1, 16)  ParameterScaling=2^0  OutDataType=fixdt(1, 16)  OutScaling=2^0
  Gain24 : Gain  Gain=K_ret(1,5)  ParameterDataType=fixdt(1, 16)  ParameterScaling=2^0  OutDataType=fixdt(1, 16)  OutScaling=2^0
  Gain25 : Gain  Gain=K_ret(1,1)  ParameterDataType=fixdt(1, 16)  ParameterScaling=2^0  OutDataType=fixdt(1, 16)  OutScaling=2^0
  Gain3 : Gain  Gain=1/128  ParameterDataType=fixdt(1, 16)  ParameterScaling=2^0  OutDataType=fixdt(1, 16)  OutScaling=2^0
  Gain32 : Gain  Gain=K_ret(2,1)  ParameterDataType=fixdt(1, 16)  ParameterScaling=2^0  OutDataType=fixdt(1, 16)  OutScaling=2^0
  Gain38 : Gain  Gain=K_ret(3,1)  ParameterDataType=fixdt(1, 16)  ParameterScaling=2^0  OutDataType=fixdt(1, 16)  OutScaling=2^0
  Gain4 : Gain  Gain=-0.938349/100  ParameterDataType=fixdt(1, 16)  ParameterScaling=2^0  OutDataType=fixdt(1, 16)  OutScaling=2^0
  Gain5 : Gain  Gain=-0.00938349  ParameterDataType=fixdt(1, 16)  ParameterScaling=2^0  OutDataType=fixdt(1, 16)  OutScaling=2^0
  Gain6 : Gain  Gain=1/128  ParameterDataType=fixdt(1, 16)  ParameterScaling=2^0  OutDataType=fixdt(1, 16)  OutScaling=2^0
  Gain7 : Gain  Gain=1/80  ParameterDataType=fixdt(1, 16)  ParameterScaling=2^0  OutDataType=fixdt(1, 16)  OutScaling=2^0
  Gain8 : Gain  Gain=K_ret(2,2)  ParameterDataType=fixdt(1, 16)  ParameterScaling=2^0  OutDataType=fixdt(1, 16)  OutScaling=2^0
  Gain9 : Gain  Gain=K_ret(3,2)  ParameterDataType=fixdt(1, 16)  ParameterScaling=2^0  OutDataType=fixdt(1, 16)  OutScaling=2^0
  KvPhi : Gain  Gain=KV(3,1)  ParameterDataType=fixdt(1, 16)  ParameterScaling=2^0  OutDataType=fixdt(1, 16)  OutScaling=2^0
  KvPhi1 : Gain  Gain=KV(3,2)  ParameterDataType=fixdt(1, 16)  ParameterScaling=2^0  OutDataType=fixdt(1, 16)  OutScaling=2^0
  KvPhi2 : Gain  Gain=KV(3,3)  ParameterDataType=fixdt(1, 16)  ParameterScaling=2^0  OutDataType=fixdt(1, 16)  OutScaling=2^0
  KvPsi : Gain  Gain=KV(1,1)  ParameterDataType=fixdt(1, 16)  ParameterScaling=2^0  OutDataType=fixdt(1, 16)  OutScaling=2^0
  KvPsi1 : Gain  Gain=KV(1,2)  ParameterDataType=fixdt(1, 16)  ParameterScaling=2^0  OutDataType=fixdt(1, 16)  OutScaling=2^0
  KvPsi2 : Gain  Gain=KV(1,3)  ParameterDataType=fixdt(1, 16)  ParameterScaling=2^0  OutDataType=fixdt(1, 16)  OutScaling=2^0
  KvTheta : Gain  Gain=KV(2,1)  ParameterDataType=fixdt(1, 16)  ParameterScaling=2^0  OutDataType=fixdt(1, 16)  OutScaling=2^0
  KvTheta1 : Gain  Gain=KV(2,2)  ParameterDataType=fixdt(1, 16)  ParameterScaling=2^0  OutDataType=fixdt(1, 16)  OutScaling=2^0
  KvTheta2 : Gain  Gain=KV(2,3)  ParameterDataType=fixdt(1, 16)  ParameterScaling=2^0  OutDataType=fixdt(1, 16)  OutScaling=2^0
  Mux : Mux
  Saturation : Saturate  UpperLimit=255  LowerLimit=0  OutDataType=fixdt(1, 16)  OutScaling=2^0
  Sum{1,7,12,15} (4 alike) : Sum  Inputs=+++  OutDataType=fixdt(1, 16)  OutScaling=2^0
  Sum{3,10,16,18..20,23..24,32} (9 alike) : Sum  Inputs=++|  OutDataType=fixdt(1, 16)  OutScaling=2^0
  Sum{2,4,9,11,13..14} (6 alike) : Sum  Inputs=+-  OutDataType=fixdt(1, 16)  OutScaling=2^0
  Sum17 : Sum  Inputs=|+-  OutDataType=fixdt(1, 16)  OutScaling=2^0
  Sum21 : Sum  Inputs=-+|  OutDataType=fixdt(1, 16)  OutScaling=2^0
  Sum22 : Sum  Inputs=|+-  OutDataType=fixdt(1, 16)  OutScaling=2^0
  Sum25 : Sum  Inputs=|+-  OutDataType=fixdt(1, 16)  OutScaling=2^0
  Sum26 : Sum  Inputs=-+|  OutDataType=fixdt(1, 16)  OutScaling=2^0
  Sum33 : Sum  Inputs=-+|  OutDataType=fixdt(1, 16)  OutScaling=2^0
  Sum5 : Sum  Inputs=+-+  OutDataType=fixdt(1, 16)  OutScaling=2^0
  Sum6 : Sum  Inputs=++-  OutDataType=fixdt(1, 16)  OutScaling=2^0
  Sum8 : Sum  Inputs=+--  OutDataType=fixdt(1, 16)  OutScaling=2^0
  Out1 : Outport  OutDataType=fixdt(1, 16)  OutScaling=2^0
  wires:
  Saturation/1 -> Out1/1
  Mux/1 -> Saturation/1
  [thrust_set] -> Sum8/1, Sum7/1, Sum6/1, Sum5/1
  Sum25/1 -> Sum6/2, Sum8/2  "m_phi"
  Sum6/1 -> Mux/2  "M2"
  Sum7/1 -> Mux/3  "M3"
  Sum8/1 -> Mux/4  "M4"
  Sum5/1 -> Mux/1  "M1"
  Gain1/1 -> [phi]
  Gain/1 -> [theta]
  Demux/9 -> [thrust_set]
  Demux/1 -> Gain/1
  Demux/2 -> Gain1/1
  In1/1 -> Demux/1
  Demux/10 -> [vx]
  Demux/11 -> [vy]
  Demux/12 -> [rpsi]
  Sum17/1 -> Sum5/3, Sum6/3, Sum7/3, Sum8/3  "m_psi"
  [phi_set] -> KvPhi/1, KvPhi1/1, KvPhi2/1
  [rpsi_set] -> KvPsi/1, KvPsi2/1, KvPsi1/1
  Demux/3 -> Sum4/1
  Sum4/1 -> Gain2/1
  Constant2/1 -> Sum4/2, Sum9/2, Sum14/2
  Gain2/1 -> [r_phi]
  Demux/4 -> Sum9/1
  Sum9/1 -> Gain4/1
  Gain4/1 -> [r_theta]
  Gain5/1 -> [r_psi]
  Demux/5 -> Sum14/1
  Sum14/1 -> Gain5/1
  KvPsi/1 -> Sum12/1
  KvTheta/1 -> Sum12/2
  KvPhi/1 -> Sum12/3
  KvPsi1/1 -> Sum1/1
  KvTheta1/1 -> Sum1/2
  KvPhi1/1 -> Sum1/3
  KvPhi2/1 -> Sum15/3
  KvTheta2/1 -> Sum15/2
  KvPsi2/1 -> Sum15/1
  [theta_set] -> KvTheta/1, KvTheta1/1, KvTheta2/1
  Gain3/1 -> [phi_set]
  Demux/6 -> Sum2/1
  Sum2/1 -> Gain3/1
  Constant1/1 -> Sum2/2, Sum13/2, Sum11/2
  Gain7/1 -> [rpsi_set]
  Gain6/1 -> [theta_set]
  Sum11/1 -> Gain6/1
  Sum13/1 -> Gain7/1
  Demux/8 -> Sum13/1
  Demux/7 -> Sum11/1
  Gain8/1 -> Sum23/1
  Sum24/1 -> Sum23/2
  Sum23/1 -> Sum3/2
  Sum26/1 -> Sum24/2
  Gain23/1 -> Sum26/2
  Sum32/1 -> Sum10/2
  Sum10/1 -> Sum16/2
  Sum33/1 -> Sum32/2
  Gain19/1 -> Sum26/1
  Gain13/1 -> Sum24/1
  Gain32/1 -> Sum3/1
  Gain38/1 -> Sum16/1
  Gain9/1 -> Sum10/1
  Gain10/1 -> Sum32/1
  Gain14/1 -> Sum33/1
  Gain15/1 -> Sum33/2
  Gain25/1 -> Sum18/1
  Sum20/1 -> Sum19/2
  Sum19/1 -> Sum18/2
  Sum21/1 -> Sum20/2
  Gain24/1 -> Sum21/2
  Gain22/1 -> Sum21/1
  Gain21/1 -> Sum20/1
  Gain20/1 -> Sum19/1
  [r_psi] -> Gain25/1, Gain32/1, Gain38/1
  [theta] -> Gain20/1, Gain8/1, Gain9/1
  [phi] -> Gain21/1, Gain13/1, Gain10/1
  [r_phi] -> Gain22/1, Gain19/1, Gain14/1
  [r_theta] -> Gain24/1, Gain23/1, Gain15/1
  Sum12/1 -> Sum17/1
  Sum18/1 -> Sum17/2
  Sum1/1 -> Sum22/1
  Sum3/1 -> Sum22/2
  Sum22/1 -> Sum7/2, Sum5/2  "m_theta"
  Sum16/1 -> Sum25/2  "Phi_Back"
  Sum15/1 -> Sum25/1

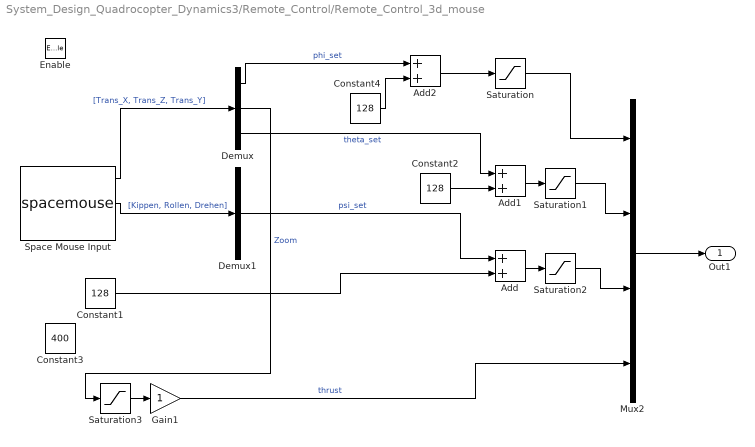
== system System_Design_Quadrocopter_Dynamics3/Remote_Control/Remote_Control_3d_mouse ==
  Enable : EnablePort  PropagateVarSize=During execution
  Add : Sum
  Add1 : Sum
  Add2 : Sum
  Constant1 : Constant  Value=128
  Constant2 : Constant  Value=128
  Constant3 : Constant  Value=400
  Constant4 : Constant  Value=128
  Demux : Demux  Outputs=3
  Demux1 : Demux  Outputs=3
  Gain1 : Gain
  Mux2 : Mux
  Saturation : Saturate  UpperLimit=255  LowerLimit=0
  Saturation1 : Saturate  UpperLimit=255  LowerLimit=0
  Saturation2 : Saturate  UpperLimit=255  LowerLimit=0
  Saturation3 : Saturate  UpperLimit=inf  LowerLimit=0
  Space Mouse Input : S-Function  AncestorBlock=vrlib/Space Mouse Input  FunctionName=spacemouse  Parameters=Port, OutputType, InitialPosition, InitialRotation, PositionSensitivity, RotationSensitivity, Dominant, NormalizeAngle, DisableTranslation, DisableRotation, PositionLow, PositionUp, EnableLimit  EnableBusSupport=off  mask(Space Mouse Input){Port=USB1, OutputType=Speed, Dominant=off, DisableTranslation=off, DisableRotation=off, NormalizeAngle=off, EnableLimit=on, PositionSensitivity=15, RotationSensitivity=15, InitialPosition=[0 0 0], InitialRotation=[0 0 0], PositionLow=[0 0 0], PositionUp=[255 255 255]}
      mask prompts: OutputType "Output type:"; Dominant "Dominant mode"; DisableTranslation "Disable position movement"; DisableRotation "Disable rotation movement"; NormalizeAngle "Normalize output angle"; EnableLimit "Limit position"; PositionSensitivity "Position sensitivity:"; RotationSensitivity "Rotation sensitivity:"; InitialPosition "Initial position:"; InitialRotation "Initial rotation:"; PositionLow "Lower position limit:"; PositionUp "Upper position limit:"
      mask help: Space Mouse input device driver.
      mask Help: helpview(fullfile(docroot, 'toolbox', 'sl3d', 'sl3d.map'), 'vr_magellanspacemouse');
      mask StyleString: popup(COM1|COM2|COM3|COM4|USB1|USB2|USB3|USB4|USB),popup(Speed|Position|Viewpoint coordinates),checkbox,checkbox,checkbox,checkbox,checkbox,edit,edit,edit,edit,edit,edit
      mask CallbackString: spacemousemask|spacemousemask|||||spacemousemask||||||
      mask Display:
      | image(imread('spacemouseicon.png'))
      | port_label('output', 1, 'Translation')
      | port_label('output', 2, 'Rotation')
      | port_label('output', 3, 'Buttons')
  Out1 : Outport
  wires:
  Demux/1 -> Add2/1  "phi_set"
  Constant4/1 -> Add2/2
  Demux/3 -> Add1/1  "theta_set"
  Constant2/1 -> Add1/2
  Add/1 -> Saturation2/1
  Demux1/2 -> Add/1  "psi_set"
  Constant1/1 -> Add/2
  Space Mouse Input/2 -> Demux1/1  "[Kippen, Rollen, Drehen]"
  Space Mouse Input/1 -> Demux/1  "[Trans_X, Trans_Z, Trans_Y]"
  Gain1/1 -> Mux2/4  "thrust"
  Mux2/1 -> Out1/1
  Add2/1 -> Saturation/1
  Add1/1 -> Saturation1/1
  Saturation1/1 -> Mux2/2
  Saturation2/1 -> Mux2/3
  Saturation/1 -> Mux2/1
  Saturation3/1 -> Gain1/1
  Demux/2 -> Saturation3/1  "Zoom"

== system System_Design_Quadrocopter_Dynamics3/Remote_Control/Remote_Control_Pitch_stimuli1 ==
  Constant : Constant  Value=128  OutDataType=fixdt(1, 16)  OutScaling=2^0
  Constant1 : Constant  Value=80  OutDataType=fixdt(1, 16)  OutScaling=2^0
  Constant2 : Constant  Value=128  OutDataType=fixdt(1, 16)  OutScaling=2^0
  Constant3 : Constant  Value=128  OutDataType=fixdt(1, 16)  OutScaling=2^0
  Gain : Gain  ParameterDataType=fixdt(1, 16)  ParameterScaling=2^0  OutDataType=fixdt(1, 16)  OutScaling=2^0
  Mux1 : Mux
  Out : Outport  OutDataType=fixdt(1, 16)  OutScaling=2^0
  wires:
  Constant2/1 -> Mux1/3  "rpsi_set"
  Constant/1 -> Gain/1  "thrust"
  Mux1/1 -> Out/1
  Gain/1 -> Mux1/4  "thrust"
  Constant1/1 -> Mux1/1  "theta_set"
  Constant3/1 -> Mux1/2  "phi_set"

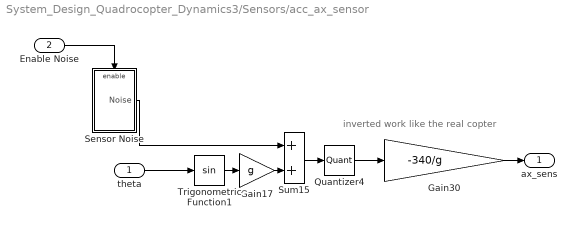
== system System_Design_Quadrocopter_Dynamics3/Sensors/acc_ax_sensor ==
  note: inverted work like the real copter
  theta : Inport
  Enable Noise : Inport  Port=2
  Gain17 : Gain  Gain=g
  Gain30 : Gain  Gain=-340/g
  Quantizer4 : Quantizer  QuantizationInterval=g/340  SampleTime=Ts
  Sensor Noise : Subsystem
  Sum15 : Sum
  Trigonometric Function1 : Trigonometry
  ax_sens : Outport
  wires:
  Sensor Noise/1(Noise) -> Sum15/1
  Sum15/1 -> Quantizer4/1
  Trigonometric Function1/1 -> Gain17/1
  Gain17/1 -> Sum15/2
  Quantizer4/1 -> Gain30/1
  theta/1 -> Trigonometric Function1/1
  Gain30/1 -> ax_sens/1
  Enable Noise/1 -> Sensor Noise/Enable

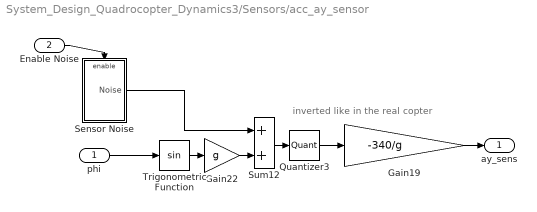
== system System_Design_Quadrocopter_Dynamics3/Sensors/acc_ay_sensor ==
  note: inverted like in the real copter
  phi : Inport
  Enable Noise : Inport  Port=2
  Gain19 : Gain  Gain=-340/g
  Gain22 : Gain  Gain=g
  Quantizer3 : Quantizer  QuantizationInterval=g/340  SampleTime=Ts
  Sensor Noise : Subsystem
  Sum12 : Sum
  Trigonometric Function : Trigonometry
  ay_sens : Outport
  wires:
  Sum12/1 -> Quantizer3/1
  Trigonometric Function/1 -> Gain22/1
  Gain22/1 -> Sum12/2
  Quantizer3/1 -> Gain19/1
  phi/1 -> Trigonometric Function/1
  Gain19/1 -> ay_sens/1
  Enable Noise/1 -> Sensor Noise/Enable
  Sensor Noise/1(Noise) -> Sum12/1

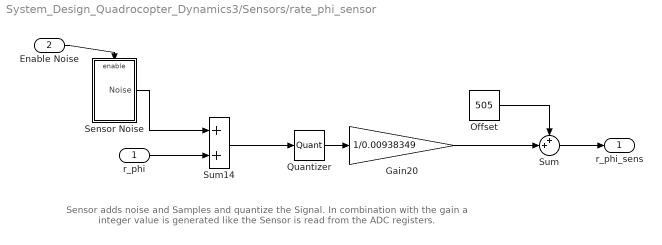
== system System_Design_Quadrocopter_Dynamics3/Sensors/rate_phi_sensor ==
  note: Sensor adds noise and Samples and quantize the Signal. In combination with the gain a integer value is generated
      | like the Sensor is read from the ADC registers.
  r_phi : Inport
  Enable Noise : Inport  Port=2
  Gain20 : Gain  Gain=1/0.00938349
  Offset : Constant  Value=505
  Quantizer : Quantizer  QuantizationInterval=0.00938349  SampleTime=Ts
  Sensor Noise : Subsystem
  Sum : Sum  Inputs=++|
  Sum14 : Sum
  r_phi_sens : Outport
  wires:
  Sum14/1 -> Quantizer/1
  Quantizer/1 -> Gain20/1
  r_phi/1 -> Sum14/2
  Gain20/1 -> Sum/2
  Offset/1 -> Sum/1
  Sum/1 -> r_phi_sens/1
  Enable Noise/1 -> Sensor Noise/Enable
  Sensor Noise/1(Noise) -> Sum14/1

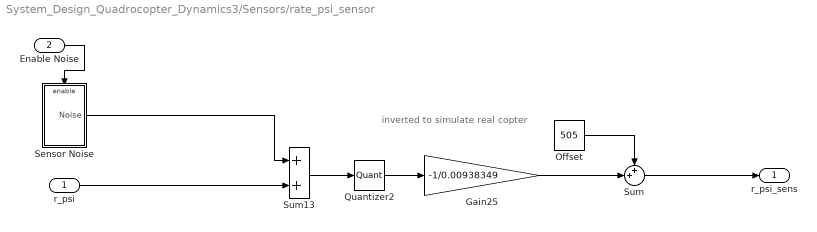
== system System_Design_Quadrocopter_Dynamics3/Sensors/rate_psi_sensor ==
  note: inverted to simulate real copter
  r_psi : Inport
  Enable Noise : Inport  Port=2
  Gain25 : Gain  Gain=-1/0.00938349
  Offset : Constant  Value=505
  Quantizer2 : Quantizer  QuantizationInterval=0.00938349  SampleTime=Ts
  Sensor Noise : Subsystem
  Sum : Sum  Inputs=++|
  Sum13 : Sum
  r_psi_sens : Outport
  wires:
  Sensor Noise/1(Noise) -> Sum13/1
  Sum13/1 -> Quantizer2/1
  Quantizer2/1 -> Gain25/1
  r_psi/1 -> Sum13/2
  Offset/1 -> Sum/1
  Gain25/1 -> Sum/2
  Sum/1 -> r_psi_sens/1
  Enable Noise/1 -> Sensor Noise/Enable

== system System_Design_Quadrocopter_Dynamics3/Sensors/rate_theta_sensor ==
  note: inverted to worj like in the real copter
  r_theta : Inport
  Enable Noise : Inport  Port=2
  Gain27 : Gain  Gain=-1/0.00938349
  Offset : Constant  Value=505
  Quantizer1 : Quantizer  QuantizationInterval=0.00938349  SampleTime=Ts
  Sensor Noise : Subsystem
  Sum : Sum  Inputs=++|
  Sum16 : Sum
  r_theta_sens : Outport
  wires:
  Sum16/1 -> Quantizer1/1
  Quantizer1/1 -> Gain27/1
  r_theta/1 -> Sum16/2
  Offset/1 -> Sum/1
  Gain27/1 -> Sum/2
  Sum/1 -> r_theta_sens/1
  Enable Noise/1 -> Sensor Noise/Enable
  Sensor Noise/1(Noise) -> Sum16/1

== system System_Design_Quadrocopter_Dynamics3/Sensors/acc_ax_sensor/Sensor Noise ==
  Enable : EnablePort  PropagateVarSize=During execution
  Random Number3 : RandomNumber  Variance=0.0003  Seed=676  SampleTime=Ts
  Noise : Outport
  wires:
  Random Number3/1 -> Noise/1

== system System_Design_Quadrocopter_Dynamics3/Sensors/acc_ay_sensor/Sensor Noise ==
  Enable : EnablePort  PropagateVarSize=During execution
  Random Number2 : RandomNumber  Variance=0.0003  Seed=4564  SampleTime=0.01
  Noise : Outport
  wires:
  Random Number2/1 -> Noise/1

== system System_Design_Quadrocopter_Dynamics3/Sensors/rate_phi_sensor/Sensor Noise ==
  Enable : EnablePort  PropagateVarSize=During execution
  Random Number1 : RandomNumber  Variance=3.0462e-8  Seed=45632  SampleTime=0.01
  Noise : Outport
  wires:
  Random Number1/1 -> Noise/1

== system System_Design_Quadrocopter_Dynamics3/Sensors/rate_psi_sensor/Sensor Noise ==
  Enable : EnablePort  PropagateVarSize=During execution
  Random Number4 : RandomNumber  Variance=3.0462e-8  Seed=1634  SampleTime=0.01
  Noise : Outport
  wires:
  Random Number4/1 -> Noise/1

== system System_Design_Quadrocopter_Dynamics3/Sensors/rate_theta_sensor/Sensor Noise ==
  Enable : EnablePort  PropagateVarSize=During execution
  Random Number5 : RandomNumber  Variance=3.0462e-8  Seed=4731  SampleTime=0.01
  Noise : Outport
  wires:
  Random Number5/1 -> Noise/1
